simulink model "sim_topic1"  (R2023b)
settings: Solver=VariableStepAuto  StartTime=0.0  StopTime=N  RelTol=1e-3
undefined symbols (not defined in the file): Ad, Bd, T, xd0
settings Model: Creator=user  LastModifiedBy=user

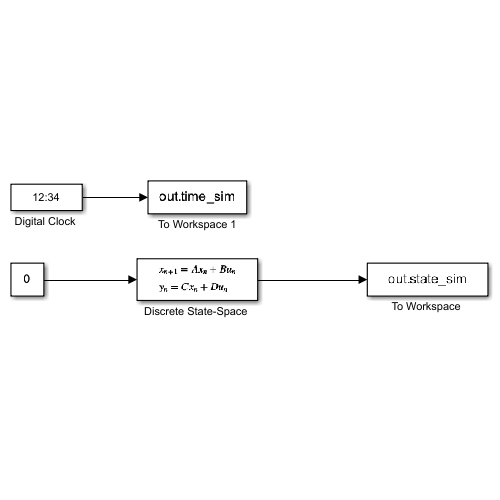
[thumbnail: Simulink's stored preview of the top-level diagram]
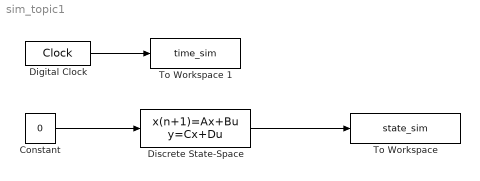
== system sim_topic1 ==
  Constant : Constant  Value=0  SampleTime=T
  "Digital Clock " : DigitalClock  SampleTime=T
  "Discrete State-Space " : DiscreteStateSpace  A=Ad  B=Bd  C=eye(2)  D=zeros(2,1)  InitialCondition=xd0  SampleTime=T
  "To Workspace " : ToWorkspace  VariableName=state_sim  SampleTime=T
  To Workspace 1 : ToWorkspace  VariableName=time_sim  SampleTime=-1
  wires:
  Constant/1 -> "Discrete State-Space "/1
  "Discrete State-Space "/1 -> "To Workspace "/1
  "Digital Clock "/1 -> To Workspace 1/1
